simulink model "Model2"  (R2017a)
settings: Solver=ode23t  StartTime=0.0  StopTime=10.0  RelTol=1e-4
values from neighbouring files (symbols this model uses):
  param = evalin('base','param')    [getSaveInfo.m]    (also in loadBackUp.m)
(part 3 of 3)

== matlab function Model2/PodwojnyIntegrator/kinematyka ==
  data: q input; qp input; z input; zp input; k output; kp output; kpp output
function [k,kp,kpp] = fcn(q,qp,z,zp)

c1=cos(q(6));
c3=cos(q(8));
s1=sin(q(6));
s3=sin(q(8));
c01=cos(q(3)+q(6));
s01=sin(q(3)+q(6));
c0=cos(q(3));
s0=sin(q(3));

k=[q(1)+(1/5).*cos(q(3))+(1/10).*(3+2.*c3).*cos(q(3)+q(6));
   q(2)+(1/5).*sin(q(3))+(1/10).*(3+2.*c3).*sin(q(3)+q(6));
  (1/10).*(2.*cos(q(3))+(3+2.*c3).*cos(q(3)+q(6)));
  (1/10).*(2.*sin(q(3))+(3+2.*c3).*sin(q(3)+q(6)));
  q(7)+s3];

Phi=[c0+(-2/3).*s0+(-1/3).*(3+2.*c3).*s01,c0+(1/3).*(2.*s0+(3+2.*c3).* ...
  s01),(-1/10).*(3+2.*c3).*s01,0,(-1/5).*c01.*s3;(2/3).*c0+c01.*(1+( ...
  2/3).*c3)+s0,(-2/3).*c0+(-1/3).*c01.*(3+2.*c3)+s0,(1/10).*c01.*(3+ ...
  2.*c3),0,(-1/5).*s01.*s3;0,0,(-1/10).*(3+2.*c3).*s01,0,(-1/5).* ...
  c01.*s3;0,0,(1/10).*c01.*(3+2.*c3),0,(-1/5).*s01.*s3;0,0,0,1,c3]; ...
  
Phip=[(1/3).*((-1).*c01.*(3+2.*c3).*qp(6)+(-1).*qp(3).*(2.*c0+c01.*(3+2.* ...
  c3)+3.*s0)+2.*qp(8).*s01.*s3),(1/3).*(c01.*(3+2.*c3).*qp(6)+qp(3).*(2.* ...
  c0+c01.*(3+2.*c3)+(-3).*s0)+(-2).*qp(8).*s01.*s3),(1/10).*((-1).* ...
  c01.*(3+2.*c3).*(qp(3)+qp(6))+2.*qp(8).*s01.*s3),0,(1/5).*((-1).*c01.* ...
  c3.*qp(8)+(qp(3)+qp(6)).*s01.*s3);c0.*qp(3)+(1/3).*((-2).*qp(3).*s0+(-1).*( ...
  3+2.*c3).*(qp(3)+qp(6)).*s01+(-2).*c01.*qp(8).*s3),(1/3).*(qp(3).*(3.*c0+ ...
  2.*s0)+(3+2.*c3).*(qp(3)+qp(6)).*s01+2.*c01.*qp(8).*s3),(1/10).*((-1).*( ...
  3+2.*c3).*(qp(3)+qp(6)).*s01+(-2).*c01.*qp(8).*s3),0,(-1/5).*c3.*qp(8).* ...
  s01+(-1/5).*c01.*(qp(3)+qp(6)).*s3;0,0,(1/10).*((-1).*c01.*(3+2.*c3).* ...
  (qp(3)+qp(6))+2.*qp(8).*s01.*s3),0,(1/5).*((-1).*c01.*c3.*qp(8)+(qp(3)+qp(6)) ...
  .*s01.*s3);0,0,(1/10).*((-1).*(3+2.*c3).*(qp(3)+qp(6)).*s01+(-2).* ...
  c01.*qp(8).*s3),0,(-1/5).*c3.*qp(8).*s01+(-1/5).*c01.*(qp(3)+qp(6)).*s3;0, ...
  0,0,0,(-1).*qp(8).*s3];

kp=Phi*z;
kpp=Phip*z+Phi*zp;

== matlab function Model2/PodwojnyIntegrator/ObiektOdsprzegniety/zeta2v ==
  data: zeta input; q input; qp input; z input; v output
function v = fcn(zeta,q,qp,z)

c1=cos(q(6));
c3=cos(q(8));
s1=sin(q(6));
s3=sin(q(8));
c01=cos(q(3)+q(6));
s01=sin(q(3)+q(6));
c0=cos(q(3));
s0=sin(q(3));

Phi=[c0+(-2/3).*s0+(-1/3).*(3+2.*c3).*s01,c0+(1/3).*(2.*s0+(3+2.*c3).* ...
  s01),(-1/10).*(3+2.*c3).*s01,0,(-1/5).*c01.*s3;(2/3).*c0+c01.*(1+( ...
  2/3).*c3)+s0,(-2/3).*c0+(-1/3).*c01.*(3+2.*c3)+s0,(1/10).*c01.*(3+ ...
  2.*c3),0,(-1/5).*s01.*s3;0,0,(-1/10).*(3+2.*c3).*s01,0,(-1/5).* ...
  c01.*s3;0,0,(1/10).*c01.*(3+2.*c3),0,(-1/5).*s01.*s3;0,0,0,1,c3]; ...
  
Phip=[(1/3).*((-1).*c01.*(3+2.*c3).*qp(6)+(-1).*qp(3).*(2.*c0+c01.*(3+2.* ...
  c3)+3.*s0)+2.*qp(8).*s01.*s3),(1/3).*(c01.*(3+2.*c3).*qp(6)+qp(3).*(2.* ...
  c0+c01.*(3+2.*c3)+(-3).*s0)+(-2).*qp(8).*s01.*s3),(1/10).*((-1).* ...
  c01.*(3+2.*c3).*(qp(3)+qp(6))+2.*qp(8).*s01.*s3),0,(1/5).*((-1).*c01.* ...
  c3.*qp(8)+(qp(3)+qp(6)).*s01.*s3);c0.*qp(3)+(1/3).*((-2).*qp(3).*s0+(-1).*( ...
  3+2.*c3).*(qp(3)+qp(6)).*s01+(-2).*c01.*qp(8).*s3),(1/3).*(qp(3).*(3.*c0+ ...
  2.*s0)+(3+2.*c3).*(qp(3)+qp(6)).*s01+2.*c01.*qp(8).*s3),(1/10).*((-1).*( ...
  3+2.*c3).*(qp(3)+qp(6)).*s01+(-2).*c01.*qp(8).*s3),0,(-1/5).*c3.*qp(8).* ...
  s01+(-1/5).*c01.*(qp(3)+qp(6)).*s3;0,0,(1/10).*((-1).*c01.*(3+2.*c3).* ...
  (qp(3)+qp(6))+2.*qp(8).*s01.*s3),0,(1/5).*((-1).*c01.*c3.*qp(8)+(qp(3)+qp(6)) ...
  .*s01.*s3);0,0,(1/10).*((-1).*(3+2.*c3).*(qp(3)+qp(6)).*s01+(-2).* ...
  c01.*qp(8).*s3),0,(-1/5).*c3.*qp(8).*s01+(-1/5).*c01.*(qp(3)+qp(6)).*s3;0, ...
  0,0,0,(-1).*qp(8).*s3];

v=inv(Phi)*(-Phip*z+zeta)

== matlab function Model2/PodwojnyIntegrator/ObiektOdsprzegniety/v2u ==
  data: v input; q input; qp input; z input; u output
function u = fcn(v,q,qp,z)

c1=cos(q(6));
c3=cos(q(8));
s1=sin(q(6));
s3=sin(q(8));

C=[(-10/3).*c1.*(9+2.*c3).*qp(6)+(20/3).*qp(8).*s1.*s3+(100/9).*(qp(6).*(( ...
  -9/5).*s1+(-2/5).*c3.*s1)+(-1).*qp(8).*((3/5).*s3+(2/5).*c1.*s3+( ...
  4/15).*c3.*s3)),(20/3).*(8+c1.*(9+2.*c3)).*qp(3)+(10/3).*c1.*(9+2.* ...
  c3).*qp(6)+(-20/3).*qp(8).*s1.*s3+(-100/9).*(qp(6).*((-9/5).*s1+(-2/5).* ...
  c3.*s1)+(-1).*qp(8).*((3/5).*s3+(2/5).*c1.*s3+(4/15).*c3.*s3)),(-1) ...
  .*c1.*(9+2.*c3).*(qp(3)+qp(6))+2.*qp(8).*s1.*s3+(10/3).*((qp(3)+qp(6)).*(( ...
  -9/5).*s1+(-2/5).*c3.*s1)+(-1).*qp(8).*((2/5).*c1.*s3+(4/15).*c3.* ...
  s3)),0,(-2).*c1.*c3.*qp(8)+2.*(qp(3)+qp(6)).*s1.*s3+(10/3).*((-2/5).* ...
  c3.*qp(8).*s1+(-1).*qp(6).*((2/5).*c1.*s3+(4/15).*c3.*s3)+(-1).*qp(3).*( ...
  (3/5).*s3+(2/5).*c1.*s3+(4/15).*c3.*s3));(-20/3).*(8+c1.*(9+2.*c3) ...
  ).*qp(3)+(-10/3).*c1.*(9+2.*c3).*qp(6)+(20/3).*qp(8).*s1.*s3+(-100/9).*( ...
  qp(6).*((-9/5).*s1+(-2/5).*c3.*s1)+(-1).*qp(8).*((3/5).*s3+(2/5).*c1.* ...
  s3+(4/15).*c3.*s3)),(10/3).*c1.*(9+2.*c3).*qp(6)+(-20/3).*qp(8).*s1.* ...
  s3+(100/9).*(qp(6).*((-9/5).*s1+(-2/5).*c3.*s1)+(-1).*qp(8).*((3/5).* ...
  s3+(2/5).*c1.*s3+(4/15).*c3.*s3)),(-1).*c1.*(9+2.*c3).*(qp(3)+qp(6))+ ...
  2.*qp(8).*s1.*s3+(-10/3).*((qp(3)+qp(6)).*((-9/5).*s1+(-2/5).*c3.*s1)+( ...
  -1).*qp(8).*((2/5).*c1.*s3+(4/15).*c3.*s3)),0,(-2).*c1.*c3.*qp(8)+2.*( ...
  qp(3)+qp(6)).*s1.*s3+(-10/3).*((-2/5).*c3.*qp(8).*s1+(-1).*qp(6).*((2/5).* ...
  c1.*s3+(4/15).*c3.*s3)+(-1).*qp(3).*((3/5).*s3+(2/5).*c1.*s3+(4/15) ...
  .*c3.*s3));(10/3).*(qp(3).*((9/5).*s1+(2/5).*c3.*s1)+(-4/75).*c3.* ...
  qp(8).*s3),(-10/3).*(qp(3).*((9/5).*s1+(2/5).*c3.*s1)+(-4/75).*c3.* ...
  qp(8).*s3),qp(8).*((-3/5).*s3+(-4/15).*c3.*s3),0,(-4/15).*c3.*qp(3).*s3+ ...
  qp(6).*((-3/5).*s3+(-4/15).*c3.*s3);0,0,0,0,(-2).*qp(8).*s3;(10/3).*(( ...
  4/75).*c3.*qp(6).*s3+qp(3).*((3/5).*s3+(2/5).*c1.*s3+(4/15).*c3.*s3)), ...
  (-10/3).*((4/75).*c3.*qp(6).*s3+qp(3).*((3/5).*s3+(2/5).*c1.*s3+(4/15) ...
  .*c3.*s3)),(4/15).*c3.*qp(3).*s3+(-1).*qp(6).*((-3/5).*s3+(-4/15).* ...
  c3.*s3),0,0];
D=[0;0;0;0.392400000000000000E3;0.196200000000000000E2.*c3];
B=[0.266666666666666667E2,0,0,0,0;
    0,0.266666666666666667E2,0,0,0;
    0,0,1,0,0;0,0,0,1,0;0,0,0,0,1];
Q=[0.247589583333333333E3+(100/9).*(4+(18/5).*c1+(6/5).*c3+(4/5).* ...
  c1.*c3+(4/15).*c3.^2)+(-20/3).*(9+2.*c3).*s1, ...
  0.604104166666666667E2+(-100/9).*(4+(18/5).*c1+(6/5).*c3+(4/5).* ...
  c1.*c3+(4/15).*c3.^2),(10/3).*((12/5)+(9/5).*c1+(2/5).*c1.*c3+( ...
  4/15).*c3.^2)+(-1).*(9+2.*c3).*s1,0,(-2).*c1.*s3+(-4/3).*s1.*s3; ...
  0.604104166666666667E2+(-100/9).*(4+(18/5).*c1+(6/5).*c3+(4/5).* ...
  c1.*c3+(4/15).*c3.^2),0.247589583333333333E3+(100/9).*(4+(18/5).* ...
  c1+(6/5).*c3+(4/5).*c1.*c3+(4/15).*c3.^2)+(20/3).*(9+2.*c3).*s1,( ...
  -10/3).*((12/5)+(9/5).*c1+(2/5).*c1.*c3+(4/15).*c3.^2)+(-1).*(9+ ...
  2.*c3).*s1,0,(-2).*c1.*s3+(4/3).*s1.*s3;(10/3).*((12/5)+(9/5).*c1+ ...
  (2/5).*c1.*c3+(4/15).*c3.^2)+(-1).*(9+2.*c3).*s1,(-10/3).*((12/5)+ ...
  (9/5).*c1+(2/5).*c1.*c3+(4/15).*c3.^2)+(-1).*(9+2.*c3).*s1,(12/5)+ ...
  (6/5).*c3+(4/15).*c3.^2,0,0;0,0,0,40,2.*c3;(-2).*c1.*s3+(-4/3).* ...
  s1.*s3,(-2).*c1.*s3+(4/3).*s1.*s3,0,2.*c3,(4/15)];

u=inv(B)*(C*z+D+Q*v);
